simulink model "PID_antiwindup_feedforward"  (R2024b)
settings: Solver=ode45  StartTime=0.0  StopTime=5  RelTol=1e-3
values from neighbouring files (symbols this model uses):
  B_C = (gbox.N * mot.Ke)/drv.dcgain    [Init.m]
  F_C = mot.Req/(drv.dcgain * mot.Kt * gbox.N)    [Init.m]
  I_C = (gbox.N * mot.Req * Jeq_hat)/(drv.dcgain * mot.Kt)    [Init.m]
  Kw = 1/Tw*0.05    (= 1.66666666667)    [Init.m]
undefined symbols (not defined in the file or in its folder): Beq, gbox, Kd, Ki, Kp, rpm2rads, sens, tau_sf, tl
libraries: simulink x1
settings Model: Creator=Banaan  LastModifiedBy=lucag

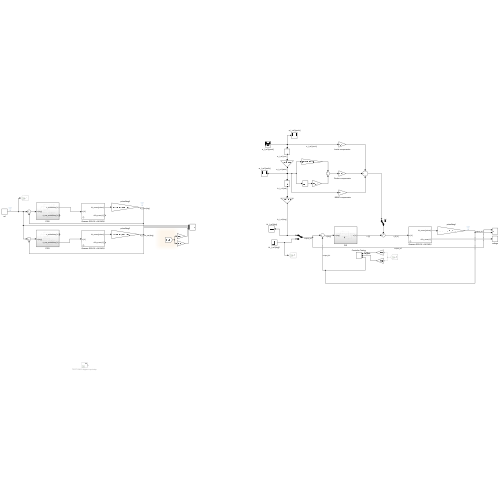
[thumbnail: Simulink's stored preview of the top-level diagram]
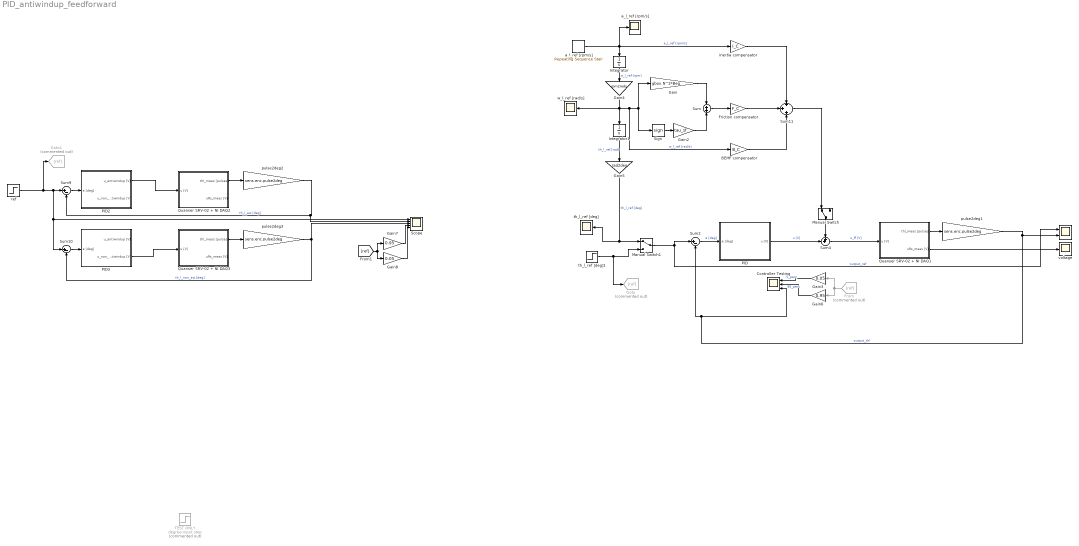
== system PID_antiwindup_feedforward ==
  " " : Scope  NumInputPorts=2
  " a_l_ref [rpm/s]" : Scope
  " th_l_ref [deg]" : Scope
  " w_l_ref [rad/s]" : Scope
  BEMF compensator : Gain  Gain=B_C
  Controller Testing : Scope  NumInputPorts=3
  Friction compensator : Gain  Gain=F_C
  From : From  Commented=on  GotoTag=ref
  Gain : Gain  Gain=gbox.N^2*Beq
  Gain2 : Gain  Gain=tau_sf
  Gain3 : Gain  Gain=0.05
  Gain4 : Gain  Gain=rpm2rads
  Gain5 : Gain  Gain=rad2deg
  Gain6 : Gain  Gain=0.95
  Gain7 : Gain  Gain=0.95
  Gain8 : Gain  Gain=0.05
  Goto : Goto  Commented=on  GotoTag=ref
  Goto1 : Goto  Commented=on  GotoTag=ref
  Inertia compensator : Gain  Gain=I_C
  Integrator : Integrator
  Integrator1 : Integrator
  Manual Switch : ManualSwitch
  Manual Switch1 : ManualSwitch
  PID : Subsystem
  PID2 : Subsystem
  PID3 : Subsystem
  Quanser SRV-02 + NI DAQ1 : Subsystem  mask(Quanser SRV-02 (with inertial load) + NI DAQ){Ts=0.001, fricType=Coulomb + viscous}
      mask prompts: Ts "NI DAQ Sample Time:"; fricType "Friction model"
      mask help: Quanser SRV-02 (with inertial load) + NI DAQ model.
      mask init:
      | %%  Sensors data
      | 
      | %   shunt resistor
      | sens.curr.Rs = 0.5;                         %   resistance [Ohm]   
      | sens.curr.uRs_std = 0.01;                   %   voltage noise standard dev [V]                           
      | sens.curr.uRs_var = sens.curr.uRs_std^2;	%   voltage noise variance [V^2]
      | 
      | %   Hewlett-Packard HEDS-5540#A06 optical encoder
      | sens.enc.ppr = 500*4;                       %   pulses per rotation
      | sens.enc.pulse2deg = 360/sens.enc.ppr;      %   [pulses] -> [deg]
      | sens.enc.pulse2rad = 2*pi/sens.enc.ppr;     %   [pulses] -> [rad]
      | sens.enc.deg2pulse = sens.enc.ppr/360;      %   [deg] -> [pulses]
      | sens.enc.rad2pulse = sens.enc.ppr/2/pi;     %   [rad] -> [pulses]
      | 
      | 
      | %%  Data acquisition board (daq) data
      | 
      | %   NI PCI-6221 DAC data
      | daq.dac.bits = 16;                                  %   resolution (bits)
      | daq.dac.fs   = 10;                                  %   full scale 
      | daq.dac.q    = 2*daq.dac.fs/(2^daq.dac.bits-1);     %	quantization
      | 
      | %   NI PCI-6221 ADC data
      | daq.adc.bits = 16;                                  %   resolution (bits)
      | daq.adc.fs   = 10;                                  %   full scale (as set in SLDRT Analog Input block)
      | daq.adc.q    = 2*daq.adc.fs/(2^daq.adc.bits-1);     %   quantization
      mask Help:
      | Riccardo Antonello (antonello@dei.unipd.it)
      | 
      | April 24, 2020
      | 
      | Dept. of Information Engineering, University of Padova
      mask TypeOptions fricType: Coulomb + viscous | Karnopp
  Quanser SRV-02 + NI DAQ2 : Subsystem  mask(Quanser SRV-02 (with inertial load) + NI DAQ){Ts=0.001, fricType=Coulomb + viscous}
      mask prompts: Ts "NI DAQ Sample Time:"; fricType "Friction model"
      mask help: Quanser SRV-02 (with inertial load) + NI DAQ model.
      mask init: same as PID_antiwindup_feedforward/Quanser SRV-02 + NI DAQ1
      mask Help:
      | Riccardo Antonello (antonello@dei.unipd.it)
      | 
      | April 24, 2020
      | 
      | Dept. of Information Engineering, University of Padova
      mask TypeOptions fricType: Coulomb + viscous | Karnopp
  Quanser SRV-02 + NI DAQ3 : Subsystem  mask(Quanser SRV-02 (with inertial load) + NI DAQ){Ts=0.001, fricType=Coulomb + viscous}
      mask prompts: Ts "NI DAQ Sample Time:"; fricType "Friction model"
      mask help: Quanser SRV-02 (with inertial load) + NI DAQ model.
      mask init: same as PID_antiwindup_feedforward/Quanser SRV-02 + NI DAQ1
      mask Help:
      | Riccardo Antonello (antonello@dei.unipd.it)
      | 
      | April 24, 2020
      | 
      | Dept. of Information Engineering, University of Padova
      mask TypeOptions fricType: Coulomb + viscous | Karnopp
  Scope : Scope  NumInputPorts=5
  Sign : Signum
  Sum : Sum  Inputs=+|+
  Sum10 : Sum  Inputs=|+-
  Sum11 : Sum  Inputs=+|+|+
  Sum2 : Sum  Inputs=|+-
  Sum4 : Sum  Inputs=++|
  Sum9 : Sum  Inputs=|+-
  TEST ONLY degree-input step : Step  Commented=on  After=360  SampleTime=0
  a_l_ref [rpm/s] : simulink/Sources/Repeating Sequence Stair  OutValues=[900 0 -900 -900 0 900]  tsamp=0.5  OutMin=[]  OutMax=[]  OutDataTypeStr=double  OutputDataTypeScalingMode=double  OutDataType=fixdt(0,8)  ConRadixGroup=Best Precision: Vector-wise  OutScaling=2^-12
  pulse2deg1 : Gain  Gain=sens.enc.pulse2deg
  pulse2deg2 : Gain  Gain=sens.enc.pulse2deg
  pulse2deg3 : Gain  Gain=sens.enc.pulse2deg
  ref : Step  After=360  SampleTime=0
  th_l_ref [deg]1 : Step  After=360  SampleTime=0
  voltage : Scope
  wires:
  Gain3/1 -> Controller Testing/1  "5_perc"
  Sum2/1 -> PID/1(e [deg])  "e [deg]"
  Quanser SRV-02 + NI DAQ1/1(thl_meas [pulses]) -> pulse2deg1/1
  Gain6/1 -> Controller Testing/2  "95_perc"
  Quanser SRV-02 + NI DAQ1/2(uRs_meas [V]) -> voltage/1
  pulse2deg1/1 -> Sum2/2, Controller Testing/3, " "/2  "output_thl"
  Integrator1/1 -> Gain5/1  "th_l_ref [rad]"
  Gain/1 -> Sum/1
  Sum/1 -> Friction compensator/1
  Sum4/1 -> Quanser SRV-02 + NI DAQ1/1(u [V])  "u_ff [V]"
  Sign/1 -> Gain2/1
  Gain2/1 -> Sum/2
  Integrator/1 -> Gain4/1  "w_l_ref [rpm]"
  Sum9/1 -> PID2/1(e [deg])
  PID2/1(u_antiwindup [V]) -> Quanser SRV-02 + NI DAQ2/1(u [V])
  Quanser SRV-02 + NI DAQ2/1(thl_meas [pulses]) -> pulse2deg2/1
  Quanser SRV-02 + NI DAQ3/1(thl_meas [pulses]) -> pulse2deg3/1
  Sum10/1 -> PID3/1(e [deg])
  pulse2deg2/1 -> Scope/2, Sum9/2  "th_l_aw [deg]"
  PID3/2(u_non_antiwindup [V]) -> Quanser SRV-02 + NI DAQ3/1(u [V])
  pulse2deg3/1 -> Scope/3, Sum10/2  "th_l_non_aw [deg]"
  ref/1 -> Goto1/1, Sum10/1, Scope/1, Sum9/1
  Gain4/1 -> BEMF compensator/1, Sign/1, Gain/1, Integrator1/1, " w_l_ref [rad/s]"/1  "w_l_ref [rad/s]"
  Gain5/1 -> Manual Switch1/1, " th_l_ref [deg]"/1  "th_l_ref [deg]"
  a_l_ref [rpm/s]/1 -> " a_l_ref [rpm/s]"/1, Inertia compensator/1, Integrator/1  "a_l_ref [rpm/s]"
  BEMF compensator/1 -> Sum11/3
  Friction compensator/1 -> Sum11/2
  Inertia compensator/1 -> Sum11/1
  Sum11/1 -> Manual Switch/1
  Manual Switch/1 -> Sum4/1
  Manual Switch1/1 -> " "/1, Sum2/1  "output_ref"
  th_l_ref [deg]1/1 -> Goto/1, Manual Switch1/2
  PID/1(u [V]) -> Sum4/2  "u [V]"
  From/1 -> Gain6/1, Gain3/1
  [ref] -> Gain8/1, Gain7/1
  Gain7/1 -> Scope/4
  Gain8/1 -> Scope/5

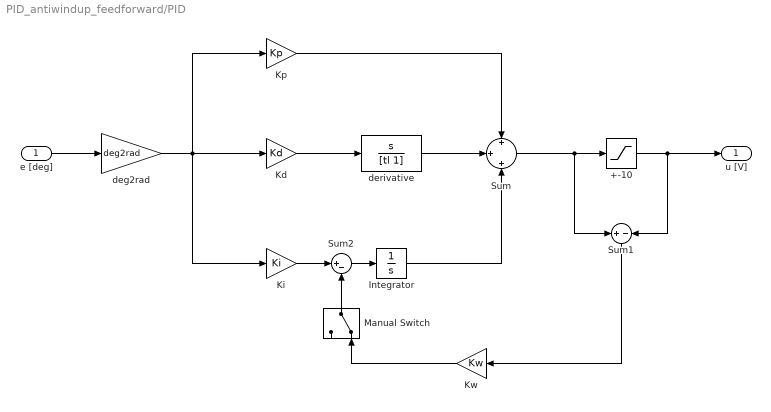
== system PID_antiwindup_feedforward/PID ==
  e [deg] : Inport
  +-10 : Saturate  UpperLimit=10  LowerLimit=-10
  Integrator : Integrator
  Kd : Gain  Gain=Kd
  Ki : Gain  Gain=Ki
  Kp : Gain  Gain=Kp
  Kw : Gain  Gain=Kw
  Manual Switch : ManualSwitch  CurrentSetting=0
  Sum : Sum  Inputs=+|+|+
  Sum1 : Sum  Inputs=+|-
  Sum2 : Sum  Inputs=|+-
  deg2rad : Gain  Gain=deg2rad
  derivative : TransferFcn  Numerator=[1 0]  Denominator=[tl 1]
  u [V] : Outport
  wires:
  e [deg]/1 -> deg2rad/1
  deg2rad/1 -> Kp/1, Ki/1, Kd/1
  Ki/1 -> Sum2/1
  Kp/1 -> Sum/1
  Integrator/1 -> Sum/3
  Kd/1 -> derivative/1
  derivative/1 -> Sum/2
  Sum/1 -> Sum1/1, +-10/1
  Sum2/1 -> Integrator/1
  Sum1/1 -> Kw/1
  +-10/1 -> u [V]/1, Sum1/2
  Manual Switch/1 -> Sum2/2
  Kw/1 -> Manual Switch/2

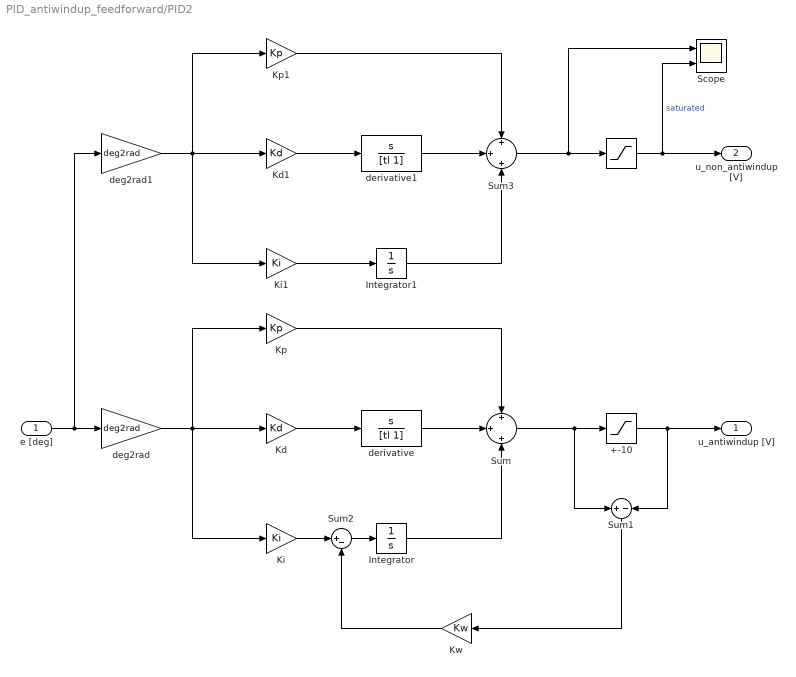
== system PID_antiwindup_feedforward/PID2 ==
  e [deg] : Inport
  " " : Saturate  UpperLimit=10  LowerLimit=-10
  +-10 : Saturate  UpperLimit=10  LowerLimit=-10
  Integrator : Integrator
  Integrator1 : Integrator
  Kd : Gain  Gain=Kd
  Kd1 : Gain  Gain=Kd
  Ki : Gain  Gain=Ki
  Ki1 : Gain  Gain=Ki
  Kp : Gain  Gain=Kp
  Kp1 : Gain  Gain=Kp
  Kw : Gain  Gain=Kw
  Scope : Scope  NumInputPorts=2
  Sum : Sum  Inputs=+|+|+
  Sum1 : Sum  Inputs=+|-
  Sum2 : Sum  Inputs=|+-
  Sum3 : Sum  Inputs=+|+|+
  deg2rad : Gain  Gain=deg2rad
  deg2rad1 : Gain  Gain=deg2rad
  derivative : TransferFcn  Numerator=[1 0]  Denominator=[tl 1]
  derivative1 : TransferFcn  Numerator=[1 0]  Denominator=[tl 1]
  u_antiwindup [V] : Outport
  u_non_antiwindup [V] : Outport  Port=2
  wires:
  " "/1 -> Scope/2, u_non_antiwindup [V]/1  "saturated"
  Integrator1/1 -> Sum3/3
  Kp1/1 -> Sum3/1
  Ki1/1 -> Integrator1/1
  Kd1/1 -> derivative1/1
  derivative1/1 -> Sum3/2
  Sum3/1 -> Scope/1, " "/1
  deg2rad1/1 -> Kd1/1, Ki1/1, Kp1/1
  +-10/1 -> Sum1/2, u_antiwindup [V]/1
  Kw/1 -> Sum2/2
  Sum1/1 -> Kw/1
  Sum2/1 -> Integrator/1
  Sum/1 -> +-10/1, Sum1/1
  derivative/1 -> Sum/2
  Kd/1 -> derivative/1
  Integrator/1 -> Sum/3
  Kp/1 -> Sum/1
  Ki/1 -> Sum2/1
  deg2rad/1 -> Kd/1, Ki/1, Kp/1
  e [deg]/1 -> deg2rad/1, deg2rad1/1

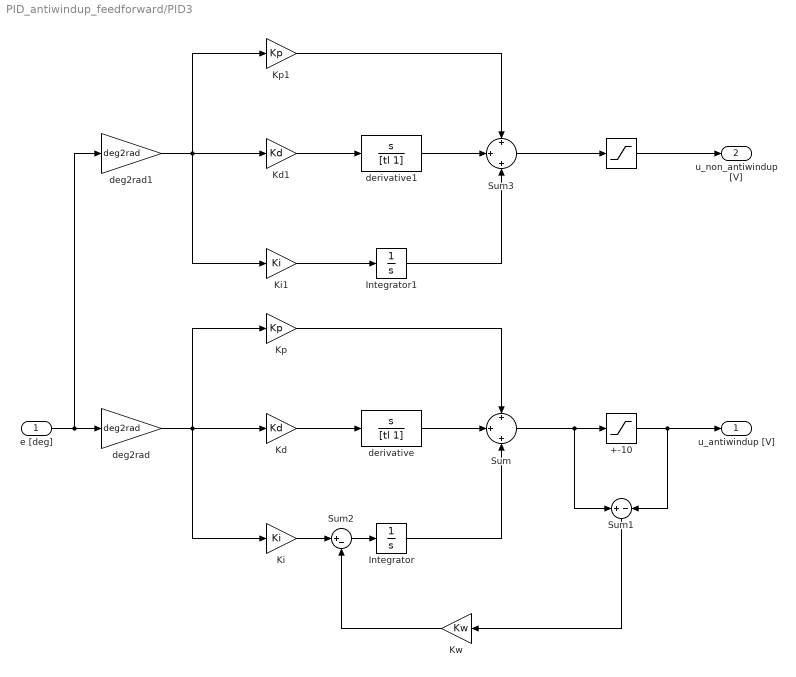
== system PID_antiwindup_feedforward/PID3 ==
  e [deg] : Inport
  " " : Saturate  UpperLimit=10  LowerLimit=-10
  +-10 : Saturate  UpperLimit=10  LowerLimit=-10
  Integrator : Integrator
  Integrator1 : Integrator
  Kd : Gain  Gain=Kd
  Kd1 : Gain  Gain=Kd
  Ki : Gain  Gain=Ki
  Ki1 : Gain  Gain=Ki
  Kp : Gain  Gain=Kp
  Kp1 : Gain  Gain=Kp
  Kw : Gain  Gain=Kw
  Sum : Sum  Inputs=+|+|+
  Sum1 : Sum  Inputs=+|-
  Sum2 : Sum  Inputs=|+-
  Sum3 : Sum  Inputs=+|+|+
  deg2rad : Gain  Gain=deg2rad
  deg2rad1 : Gain  Gain=deg2rad
  derivative : TransferFcn  Numerator=[1 0]  Denominator=[tl 1]
  derivative1 : TransferFcn  Numerator=[1 0]  Denominator=[tl 1]
  u_antiwindup [V] : Outport
  u_non_antiwindup [V] : Outport  Port=2
  wires:
  e [deg]/1 -> deg2rad1/1, deg2rad/1
  deg2rad/1 -> Kp/1, Ki/1, Kd/1
  Ki/1 -> Sum2/1
  Kp/1 -> Sum/1
  Integrator/1 -> Sum/3
  Kd/1 -> derivative/1
  derivative/1 -> Sum/2
  Sum/1 -> Sum1/1, +-10/1
  Sum2/1 -> Integrator/1
  Sum1/1 -> Kw/1
  Kw/1 -> Sum2/2
  +-10/1 -> u_antiwindup [V]/1, Sum1/2
  deg2rad1/1 -> Kp1/1, Ki1/1, Kd1/1
  Sum3/1 -> " "/1
  derivative1/1 -> Sum3/2
  Kd1/1 -> derivative1/1
  Ki1/1 -> Integrator1/1
  Kp1/1 -> Sum3/1
  Integrator1/1 -> Sum3/3
  " "/1 -> u_non_antiwindup [V]/1

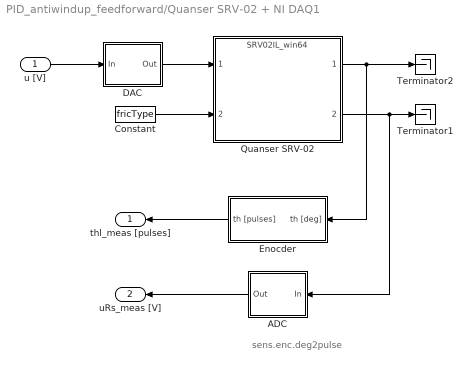
== system PID_antiwindup_feedforward/Quanser SRV-02 + NI DAQ1 ==
  note: sens.enc.deg2pulse
  u [V] : Inport
  ADC : Subsystem
  Constant : Constant  Value=fricType
  DAC : Subsystem
  Enocder : Subsystem
  Quanser SRV-02 : ModelReference  ModelNameDialog=SRV02IL_win64.slxp  ModelReferenceVersion=1.44  CopyOfModelProtected=on
  Terminator1 : Terminator
  Terminator2 : Terminator
  thl_meas [pulses] : Outport
  uRs_meas [V] : Outport  Port=2
  wires:
  Enocder/1(th [pulses]) -> thl_meas [pulses]/1
  ADC/1(Out) -> uRs_meas [V]/1
  DAC/1(Out) -> Quanser SRV-02/1
  Quanser SRV-02/2 -> ADC/1(In), Terminator1/1
  u [V]/1 -> DAC/1(In)
  Quanser SRV-02/1 -> Enocder/1(th [deg]), Terminator2/1
  Constant/1 -> Quanser SRV-02/2

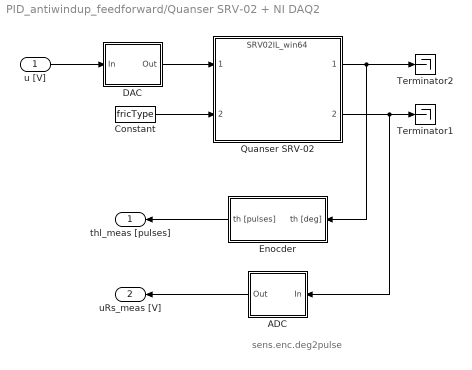
== system PID_antiwindup_feedforward/Quanser SRV-02 + NI DAQ2 ==
  note: sens.enc.deg2pulse
  u [V] : Inport
  ADC : Subsystem
  Constant : Constant  Value=fricType
  DAC : Subsystem
  Enocder : Subsystem
  Quanser SRV-02 : ModelReference  ModelNameDialog=SRV02IL_win64.slxp  ModelReferenceVersion=1.44  CopyOfModelProtected=on
  Terminator1 : Terminator
  Terminator2 : Terminator
  thl_meas [pulses] : Outport
  uRs_meas [V] : Outport  Port=2
  wires:
  Constant/1 -> Quanser SRV-02/2
  Quanser SRV-02/1 -> Terminator2/1, Enocder/1(th [deg])
  u [V]/1 -> DAC/1(In)
  Quanser SRV-02/2 -> Terminator1/1, ADC/1(In)
  DAC/1(Out) -> Quanser SRV-02/1
  ADC/1(Out) -> uRs_meas [V]/1
  Enocder/1(th [pulses]) -> thl_meas [pulses]/1

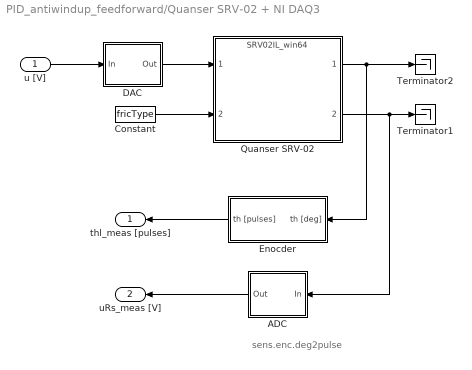
== system PID_antiwindup_feedforward/Quanser SRV-02 + NI DAQ3 ==
  note: sens.enc.deg2pulse
  u [V] : Inport
  ADC : Subsystem
  Constant : Constant  Value=fricType
  DAC : Subsystem
  Enocder : Subsystem
  Quanser SRV-02 : ModelReference  ModelNameDialog=SRV02IL_win64.slxp  ModelReferenceVersion=1.44  CopyOfModelProtected=on
  Terminator1 : Terminator
  Terminator2 : Terminator
  thl_meas [pulses] : Outport
  uRs_meas [V] : Outport  Port=2
  wires:
  Enocder/1(th [pulses]) -> thl_meas [pulses]/1
  ADC/1(Out) -> uRs_meas [V]/1
  DAC/1(Out) -> Quanser SRV-02/1
  Quanser SRV-02/2 -> ADC/1(In), Terminator1/1
  u [V]/1 -> DAC/1(In)
  Quanser SRV-02/1 -> Enocder/1(th [deg]), Terminator2/1
  Constant/1 -> Quanser SRV-02/2

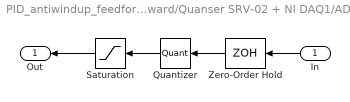
== system PID_antiwindup_feedforward/Quanser SRV-02 + NI DAQ1/ADC ==
  In : Inport
  Quantizer : Quantizer  QuantizationInterval=daq.adc.q
  Saturation : Saturate  UpperLimit=daq.adc.fs  LowerLimit=-daq.adc.fs
  Zero-Order Hold : ZeroOrderHold  SampleTime=Ts
  Out : Outport
  wires:
  Saturation/1 -> Out/1
  In/1 -> Zero-Order Hold/1
  Quantizer/1 -> Saturation/1
  Zero-Order Hold/1 -> Quantizer/1

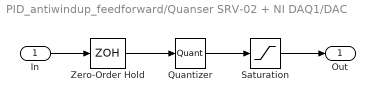
== system PID_antiwindup_feedforward/Quanser SRV-02 + NI DAQ1/DAC ==
  In : Inport
  Quantizer : Quantizer  QuantizationInterval=daq.dac.q
  Saturation : Saturate  UpperLimit=daq.dac.fs  LowerLimit=-daq.dac.fs
  Zero-Order Hold : ZeroOrderHold  SampleTime=Ts
  Out : Outport
  wires:
  Quantizer/1 -> Saturation/1
  In/1 -> Zero-Order Hold/1
  Zero-Order Hold/1 -> Quantizer/1
  Saturation/1 -> Out/1

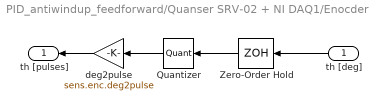
== system PID_antiwindup_feedforward/Quanser SRV-02 + NI DAQ1/Enocder ==
  th [deg] : Inport
  Quantizer : Quantizer  QuantizationInterval=sens.enc.pulse2deg
  Zero-Order Hold : ZeroOrderHold  SampleTime=Ts
  deg2pulse : Gain  Gain=sens.enc.deg2pulse
  th [pulses] : Outport
  wires:
  Quantizer/1 -> deg2pulse/1
  th [deg]/1 -> Zero-Order Hold/1
  Zero-Order Hold/1 -> Quantizer/1
  deg2pulse/1 -> th [pulses]/1

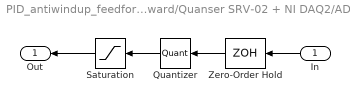
== system PID_antiwindup_feedforward/Quanser SRV-02 + NI DAQ2/ADC ==
  In : Inport
  Quantizer : Quantizer  QuantizationInterval=daq.adc.q
  Saturation : Saturate  UpperLimit=daq.adc.fs  LowerLimit=-daq.adc.fs
  Zero-Order Hold : ZeroOrderHold  SampleTime=Ts
  Out : Outport
  wires:
  Zero-Order Hold/1 -> Quantizer/1
  Quantizer/1 -> Saturation/1
  In/1 -> Zero-Order Hold/1
  Saturation/1 -> Out/1

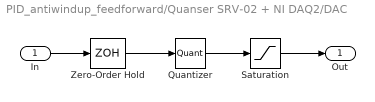
== system PID_antiwindup_feedforward/Quanser SRV-02 + NI DAQ2/DAC ==
  In : Inport
  Quantizer : Quantizer  QuantizationInterval=daq.dac.q
  Saturation : Saturate  UpperLimit=daq.dac.fs  LowerLimit=-daq.dac.fs
  Zero-Order Hold : ZeroOrderHold  SampleTime=Ts
  Out : Outport
  wires:
  Saturation/1 -> Out/1
  Zero-Order Hold/1 -> Quantizer/1
  In/1 -> Zero-Order Hold/1
  Quantizer/1 -> Saturation/1

== system PID_antiwindup_feedforward/Quanser SRV-02 + NI DAQ2/Enocder ==
  th [deg] : Inport
  Quantizer : Quantizer  QuantizationInterval=sens.enc.pulse2deg
  Zero-Order Hold : ZeroOrderHold  SampleTime=Ts
  deg2pulse : Gain  Gain=sens.enc.deg2pulse
  th [pulses] : Outport
  wires:
  deg2pulse/1 -> th [pulses]/1
  Zero-Order Hold/1 -> Quantizer/1
  th [deg]/1 -> Zero-Order Hold/1
  Quantizer/1 -> deg2pulse/1

== system PID_antiwindup_feedforward/Quanser SRV-02 + NI DAQ3/ADC ==
  In : Inport
  Quantizer : Quantizer  QuantizationInterval=daq.adc.q
  Saturation : Saturate  UpperLimit=daq.adc.fs  LowerLimit=-daq.adc.fs
  Zero-Order Hold : ZeroOrderHold  SampleTime=Ts
  Out : Outport
  wires:
  Saturation/1 -> Out/1
  In/1 -> Zero-Order Hold/1
  Quantizer/1 -> Saturation/1
  Zero-Order Hold/1 -> Quantizer/1

== system PID_antiwindup_feedforward/Quanser SRV-02 + NI DAQ3/DAC ==
  In : Inport
  Quantizer : Quantizer  QuantizationInterval=daq.dac.q
  Saturation : Saturate  UpperLimit=daq.dac.fs  LowerLimit=-daq.dac.fs
  Zero-Order Hold : ZeroOrderHold  SampleTime=Ts
  Out : Outport
  wires:
  Quantizer/1 -> Saturation/1
  In/1 -> Zero-Order Hold/1
  Zero-Order Hold/1 -> Quantizer/1
  Saturation/1 -> Out/1

== system PID_antiwindup_feedforward/Quanser SRV-02 + NI DAQ3/Enocder ==
  th [deg] : Inport
  Quantizer : Quantizer  QuantizationInterval=sens.enc.pulse2deg
  Zero-Order Hold : ZeroOrderHold  SampleTime=Ts
  deg2pulse : Gain  Gain=sens.enc.deg2pulse
  th [pulses] : Outport
  wires:
  Quantizer/1 -> deg2pulse/1
  th [deg]/1 -> Zero-Order Hold/1
  Zero-Order Hold/1 -> Quantizer/1
  deg2pulse/1 -> th [pulses]/1
